simulink model "LineFeederExercise"  (R2020b)
settings: Solver=ode45  StartTime=0.0  StopTime=100  RelTol=1e-3  EnableMultiTasking=on
undefined symbols (not defined in the file): GREEN, ORANGE, RED
settings Model: Creator=The MathWorks, Inc.  LastModifiedBy=sebastian
settings DataIOCC: LimitDataPoints=on  SaveFormat=Array  ReturnWorkspaceOutputs=off
settings OptimizationCC: ExpressionDepthLimit=2147483647  LifeSpan=1  EfficientTunableParamExpr=on
settings DebuggingCC: UnderspecifiedInitializationDetection=Classic  MergeDetectMultiDrivingBlocksExec=none  FcnCallInpInsideContextMsg=warning  StateNameClashWarn=warning  PregeneratedLibrarySubsystemCodeDiagnostic=none  SFUnexpectedBacktrackingDiag=warning  SFNoUnconditionalDefaultTransitionDiag=warning  SFExecutionAtInitializationDiag=none  ArithmeticOperatorsInVariantConditions=warning
settings HardwareCC: ProdBitPerPointer=32  ProdBitPerSizeT=32  ProdBitPerPtrDiffT=32  ProdLargestAtomicFloat=None  ProdIntDivRoundTo=Undefined  ProdEndianess=Unspecified  ProdWordSize=32  ProdHWDeviceType=32-bit Generic
settings ModelReferenceCC: PropagateSignalLabelsOutOfModel=off
settings SFSimCC: SimUseLocalCustomCode=off  MATLABDynamicMemAlloc=off  CustomCodeUndefinedFunction=UseInterfaceOnly
settings RTWCC: Description=Embedded Coder  SystemTargetFile=ert.tlc  TemplateMakefile=ert_default_tmf  RTWUseLocalCustomCode=off
settings CodeAppCC: IgnoreCustomStorageClasses=off  CustomSymbolStrType=$N$R$M  StateflowObjectComments=on  InternalIdentifier=Classic
settings ERTTargetCC: MultiwordLength=2048  GenerateSampleERTMain=on  ERTCustomFileTemplate=example_file_process.tlc  ConvertIfToSwitch=off  SuppressUnreachableDefaultCases=off
settings ConfigComp: CovMetricSettings=dw  CovSaveCumulativeToWorkspaceVar=on  CovSaveSingleToWorkspaceVar=on  CovExternalEMLEnable=off

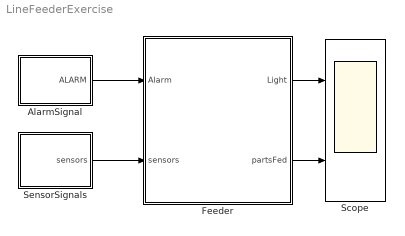
== system LineFeederExercise ==
  AlarmSignal : Subsystem
  Feeder : Stateflow chart  TreatAsAtomicUnit=on
  Scope : Scope  NumInputPorts=2
  SensorSignals : Subsystem
  wires:
  AlarmSignal/1(ALARM) -> Feeder/1(Alarm)
  SensorSignals/1(sensors) -> Feeder/2(sensors)
  Feeder/1(Light) -> Scope/1
  Feeder/2(partsFed) -> Scope/2

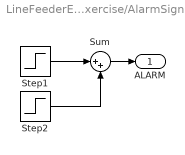
== system LineFeederExercise/AlarmSignal ==
  Step1 : Step  Time=45  SampleTime=0
  Step2 : Step  Time=80  After=-1  SampleTime=0
  Sum : Sum  Inputs=|++
  ALARM : Outport  VectorParamsAs1DForOutWhenUnconnected=off
  wires:
  Step1/1 -> Sum/1
  Step2/1 -> Sum/2
  Sum/1 -> ALARM/1

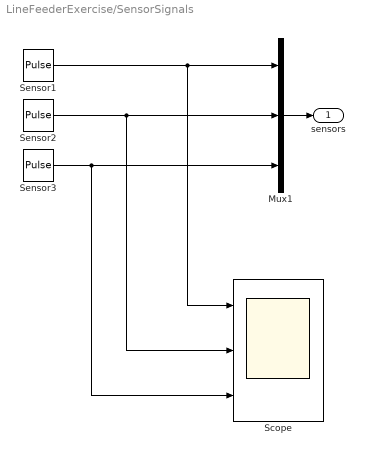
== system LineFeederExercise/SensorSignals ==
  Mux1 : Mux  Inputs=3
  Scope : Scope  NumInputPorts=3
  Sensor1 : DiscretePulseGenerator  PulseType=Time based  Amplitude=5  Period=5  PulseWidth=50  VectorParams1D=off
  Sensor2 : DiscretePulseGenerator  PulseType=Time based  Amplitude=5  Period=5  PulseWidth=80  VectorParams1D=off
  Sensor3 : DiscretePulseGenerator  PulseType=Time based  Amplitude=5  Period=5  PulseWidth=50  VectorParams1D=off
  sensors : Outport  VectorParamsAs1DForOutWhenUnconnected=off
  wires:
  Mux1/1 -> sensors/1
  Sensor1/1 -> Scope/1, Mux1/1
  Sensor2/1 -> Scope/2, Mux1/2
  Sensor3/1 -> Mux1/3, Scope/3

== stateflow chart LineFeederExercise/Feeder ==
  state InitializeSystem
    entry:
    Light = ORANGE;
  state FailState
    entry:
    Light = RED;
  state On
    entry:
    Light = GREEN;
    partsFed = 0;
    during:
    if(any(sensors >= 2))
    partsFed = partsFed + 1;
    end
  (default) -> InitializeSystem
  FailState -> InitializeSystem : [Alarm == 0]
  InitializeSystem -> FailState [order 2] : [after(5,sec)]
  InitializeSystem -> On [order 1] : [all(sensors>0)]
  On -> FailState : [Alarm == 1]
  data: Alarm input; sensors input; Light output; partsFed output; GREEN parameter; RED parameter; ORANGE parameter
